simulink model "RLS2_2_SN"  (R2024a)
settings: Solver=FixedStepAuto  StartTime=0.0  StopTime=1000  FixedStep=0.3  RelTol=1e-3
libraries: dspsrcs4 x1
settings Model: Creator=mergenelos  LastModifiedBy=mergenelos

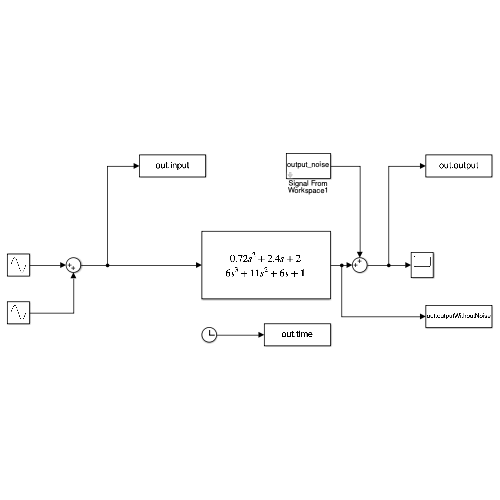
[thumbnail: Simulink's stored preview of the top-level diagram]
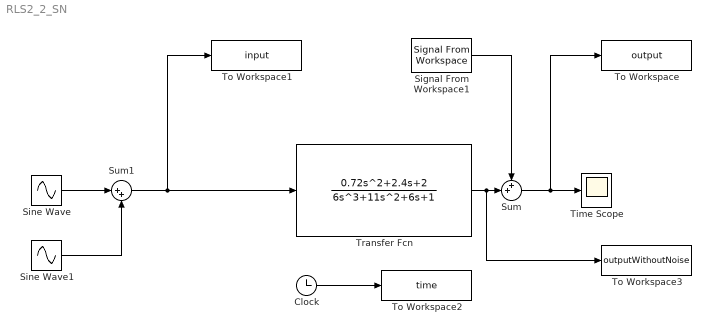
== system RLS2_2_SN ==
  Clock : Clock
  Signal From Workspace1 : dspsrcs4/Signal From Workspace  X=output_noise  Ts=0.3  nsamps=1  OutputAfterFinalValue=Setting to zero  ignoreOrWarnInputAndFrameLengths=off  OutputFrames=off
  Sine Wave : Sin  Frequency=0.1  SampleTime=0
  Sine Wave1 : Sin  Frequency=0.07  SampleTime=0
  Sum : Sum  Inputs=++|
  Sum1 : Sum  Inputs=|++
  Time Scope : Scope
  To Workspace : ToWorkspace  VariableName=output  SaveFormat=Timeseries  SampleTime=-1
  To Workspace1 : ToWorkspace  VariableName=input  SaveFormat=Timeseries  SampleTime=-1
  To Workspace2 : ToWorkspace  VariableName=time  SaveFormat=Timeseries  SampleTime=-1
  To Workspace3 : ToWorkspace  VariableName=outputWithoutNoise  SaveFormat=Timeseries  SampleTime=-1
  Transfer Fcn : TransferFcn  Numerator=[0.72 2.4 2]  Denominator=[6 11 6 1]
  wires:
  Clock/1 -> To Workspace2/1
  Sum/1 -> To Workspace/1, Time Scope/1
  Transfer Fcn/1 -> Sum/2, To Workspace3/1
  Sine Wave/1 -> Sum1/1
  Sum1/1 -> To Workspace1/1, Transfer Fcn/1
  Sine Wave1/1 -> Sum1/2
  Signal From Workspace1/1 -> Sum/1
